simulink model "double_3D_pend"  (R2023a)
settings: Solver=VariableStepAuto  StartTime=0.0  StopTime=5  MaxStep=1e-3  RelTol=1e-9  AbsTol=1e-9  EnableMultiTasking=on
InitFcn:
  | addpath quaternion_muscle\
  | data;
values from neighbouring files (symbols this model uses):
  akt = [1,1,1]    [data.m]    (also in odvozeni_svaly.m = sym('akt',[1 6]); optim_control_nlmpc.m = u'; simulation.m = [1,1,1]*0.5)
  c = 0    [data.m]    (also in neco.m = cos(0); optim_control_nlmpc.m = 100; simulation.m = 10)
  force = [1,1,0]*(-30)    [data.m]    (also in odvozeni_svaly.m = (((length / l0m)^3) * exp(8 * length / l0m - 12.9) + (exp(-(; optim_control_nlmpc.m = [1,1,1,1,1,1]*(30); simulation.m = -[1,2,1]*1)
  g = 9.81    [data.m]    (also in optim_control_nlmpc.m; simulation.m)
  IL = [8.1667, 8.1667, 1.66667,0,0,0]    [data.m]    (also in fo_python_to_matlab.m = [ILxx ILyy ILzz ILxy ILyz ILzx]; mm_python_to_matlab.m = [ILxx ILyy ILzz ILxy ILyz ILzx]; optim_control_nlmpc.m; simulation.m = [84.1667, 84.1667, 1.66667])
  initialConditions = [1,0,0,0,0,0,zeros(1,6)]*2    [data.m]    (also in simulation.m = [1,1,1,1,1,1,0,0,0,0,0,0]*0)
  IU = [8.1667, 8.1667, 1.66667,0,0,0]    [data.m]    (also in fo_python_to_matlab.m = [IUxx IUyy IUzz IUxy IUyz IUzx]; mm_python_to_matlab.m = [IUxx IUyy IUzz IUxy IUyz IUzx]; optim_control_nlmpc.m; simulation.m = [84.1667, 84.1667, 1.66667]*1e-2)
  k = 100    [data.m]    (also in neco.m = elips_pars.k; optim_control_nlmpc.m = 0; simulation.m = 1)
  l0m = [12,25,15]    [data.m]    (also in odvozeni_svaly.m = sym('l0m', [1 6]); optim_control_nlmpc.m = [30,30,30,30,30,30]; simulation.m = [10,20,10])
  m = rand(1,2)*10    [data.m]    (also in fo_python_to_matlab.m = [m1,m2]; mm_python_to_matlab.m = [m1,m2]; neco.m = elips_pars.m; optim_control_nlmpc.m = [5,10])
  rigid1C = [0,0,5]    [data.m]    (also in fo_python_to_matlab.m = [rigid1Cx, rigid1Cy, rigid1Cz]; mm_python_to_matlab.m = [rigid1Cx, rigid1Cy, rigid1Cz]; optim_control_nlmpc.m)
  rigid1P = [0,0,-5]    [data.m]    (also in fo_python_to_matlab.m = [rigid1Px, rigid1Py, rigid1Pz]; mm_python_to_matlab.m = [rigid1Px, rigid1Py, rigid1Pz]; optim_control_nlmpc.m)
  rigid2C = [0,0,5]    [data.m]    (also in fo_python_to_matlab.m = [rigid2Cx, rigid2Cy, rigid2Cz]; mm_python_to_matlab.m = [rigid2Cx, rigid2Cy, rigid2Cz]; optim_control_nlmpc.m)
  s = sin(0)    [neco.m]
undefined symbols (not defined in the file or in its folder): Ixx, Iyy, Izz, l, q1init, q2init, X, Y, Z
libraries: sm_lib x104, nesl_utility x52
(part 4 of 5)

== system double_3D_pend/Subsystem5 ==
  PS-Simulink Converter : nesl_utility/PS-Simulink Converter  PhysicalDomain=network_engine_domain  SubClassName=ps_output  LeftPortType=input  RightPortType=output  PseudoPeriodic=off  Frequencies=[]  VectorFormat=inherit  Unit=inherit  AffineConversion=off
  Spherical Joint1 : sm_lib/Joints/Spherical Joint  JointMode=Normal  SenseConstraintForce=off  SenseConstraintForceX=off  SenseConstraintForceY=off  SenseConstraintForceZ=off  SenseConstraintTorque=off  SenseConstraintTorqueX=off  SenseConstraintTorqueY=off  SenseConstraintTorqueZ=off  SenseTotalForce=off  SenseTotalForceX=off  SenseTotalForceY=off  SenseTotalForceZ=off  SenseTotalTorque=off  SenseTotalTorqueX=off  SenseTotalTorqueY=off  SenseTotalTorqueZ=off  CompositeWrenchDir=FollowerOnBase  CompositeWrenchFrame=BaseFrame  EqPosRotationMethod=None  EqPosRotationAngleUnits=deg  EqPosRotationStandardAxis=+Z  EqPosRotationAngle=0.0  EqPosRotationArbitraryAxis=[0 0 1]  EqPosFollAlignAxisA=+X  EqPosBaseAlignAxisA=+Y  EqPosFollAlignAxisB=+Y  EqPosBaseAlignAxisB=+Z  EqPosRotationSequenceAxes=FollowerAxes  EqPosRotationSequence=XYX  EqPosRotationSequenceAngles=[0 0 0]  EqPosRotationSequenceAnglesUnits=deg  EqPosRotationMatrix=[1 0 0; 0 1 0; 0 0 1]  EqPosQuaternion=[1 0 0 0]  SpringStiffness=0  SpringStiffnessUnits=N*m/deg  DampingCoefficient=c  DampingCoefficientUnits=N*m/(rad/s)  ActuateTorqueX=off  ActuateTorqueY=off  ActuateTorqueZ=off  ActuateTorque=off  TorqueActuationMode=InputTorque  MotionActuationMode=ComputedMotion  ActuationFrame=FollowerFrame  SensePosition=on  SenseVelocityX=off  SenseVelocityY=off  SenseVelocityZ=off  SenseVelocity=off  SenseAccelerationX=off  SenseAccelerationY=off  SenseAccelerationZ=off  SenseAcceleration=off  SenseTorqueX=off  SenseTorqueY=off  SenseTorqueZ=off  SenseTorqueForce=off  SenseLowerLimitTorqueMag=off  SenseUpperLimitTorqueMag=off  SensingFrame=BaseFrame  LowerLimitSpecify=off  LowerLimitBound=15  LowerLimitBoundUnits=deg  LowerLimitStiffness=1e4  LowerLimitStiffnessUnits=N*m/deg  LowerLimitDamping=10  LowerLimitDampingUnits=N*m/(deg/s)  LowerLimitTransitionRegionWidth=0.1  LowerLimitTransitionRegionWidthUnits=deg  UpperLimitSpecify=off  UpperLimitBound=45  UpperLimitBoundUnits=deg  UpperLimitStiffness=1e4  UpperLimitStiffnessUnits=N*m/deg  UpperLimitDamping=10  UpperLimitDampingUnits=N*m/(deg/s)  UpperLimitTransitionRegionWidth=0.1  UpperLimitTransitionRegionWidthUnits=deg  PositionTargetRotationMethod=Quaternion  PositionTargetRotationAngleUnits=deg  PositionTargetRotationStandardAxis=+Z  PositionTargetRotationAngle=0.0  PositionTargetRotationArbitraryAxis=[0 0 1]  PositionTargetFollAlignAxisA=+X  PositionTargetBaseAlignAxisA=+Y  PositionTargetFollAlignAxisB=+Y  PositionTargetBaseAlignAxisB=+Z  PositionTargetRotationSequenceAxes=FollowerAxes  PositionTargetRotationSequence=XYZ  PositionTargetRotationSequenceAngles=initialConditions(4:6)  PositionTargetRotationSequenceAnglesUnits=rad  PositionTargetRotationMatrix=[1 0 0; 0 1 0; 0 0 1]  PositionTargetQuaternion=q2init  PositionTargetSpecify=on  PositionTargetPriority=High  VelocityTargetValue=[0 0 0]  VelocityTargetValueUnits=deg/s  VelocityTargetSpecify=off  VelocityTargetPriority=High  VelocityTargetInFollowerFrame=on
  B : PMIOPort  Side=Left
  F : PMIOPort  Port=2  Side=Right
  Outport : Outport
  wires:
  PS-Simulink Converter/1 -> Outport/1
  connections:
  Spherical Joint1/RConn2 -- PS-Simulink Converter/LConn1
  Spherical Joint1/RConn1 -- F/RConn1
  B/RConn1 -- Spherical Joint1/LConn1

== matlab function double_3D_pend/Transform matrix ==
  data: u input; R output
function R = fcn(u)

R = zeros(3,3);

rot = xyzSeq(u(1),u(2),u(3))*xyzSeq(u(4),u(5),u(6));
R = rot(1:3,1:3);

function xyz = xyzSeq(x,y,z)
    xyz = R_x(x)*R_y(y)*R_z(z);
end
    
function rot_phix = R_x(phix)
    rot_phix = [1,0        , 0        ,0;
                0,cos(phix),-sin(phix),0;
                0,sin(phix), cos(phix),0;
                0,0        , 0        ,1];
end

function rot_phiy = R_y(phiy)
    rot_phiy = [cos(phiy),0,sin(phiy),0;
                0        ,1,0        ,0;
               -sin(phiy),0,cos(phiy),0;
                0        ,0,0        ,1];
end

function rot_phiz = R_z(phiz)
    rot_phiz = [cos(phiz),-sin(phiz),0,0;
                sin(phiz), cos(phiz),0,0;
                0           ,0      ,1,0;
                0           ,0      ,0,1];
end

end

== matlab function double_3D_pend/DELT13/Active_factor_norm ==
  data: Fa_norm output; lm input; l0 input; a input
function Fa_norm = fcn(lm,l0,a)
f_gauss = 0.25;
Fa_norm = (exp(-(lm/l0-1)^2/f_gauss))*a;

== matlab function double_3D_pend/DELT4/Active_factor_norm ==
  data: Fa_norm output; lm input; l0 input; a input
function Fa_norm = fcn(lm,l0,a)
f_gauss = 0.25;
Fa_norm = (exp(-(lm/l0-1)^2/f_gauss))*a;

== matlab function double_3D_pend/DELT4/Passive_force_norm ==
  data: lm input; Fp_norm output; l0 input
function Fp_norm = fcn(lm,l0)
Fp_norm = ((lm/l0)^3)*exp(8*lm/l0-12.9);

== matlab function double_3D_pend/DELT5/Active_factor_norm ==
  data: Fa_norm output; lm input; l0 input; a input
function Fa_norm = fcn(lm,l0,a)
f_gauss = 0.25;
Fa_norm = (exp(-(lm/l0-1)^2/f_gauss))*a;

== matlab function double_3D_pend/DELT5/Passive_force_norm ==
  data: lm input; Fp_norm output; l0 input
function Fp_norm = fcn(lm,l0)
Fp_norm = ((lm/l0)^3)*exp(8*lm/l0-12.9);

== matlab function double_3D_pend/DELT6/Active_factor_norm ==
  data: Fa_norm output; lm input; l0 input; a input
function Fa_norm = fcn(lm,l0,a)
f_gauss = 0.25;
Fa_norm = (exp(-(lm/l0-1)^2/f_gauss))*a;

== matlab function double_3D_pend/DELT6/Passive_force_norm ==
  data: lm input; Fp_norm output; l0 input
function Fp_norm = fcn(lm,l0)
Fp_norm = ((lm/l0)^3)*exp(8*lm/l0-12.9);

== matlab function double_3D_pend/MATLAB Function1 ==
  data: u input; y output
function y = fcn(u)
y = XYZ_angles(u);

== matlab function double_3D_pend/DELT10/Active_factor_norm ==
  data: Fa_norm output; lm input; l0 input; a input
function Fa_norm = fcn(lm,l0,a)
f_gauss = 0.25;
Fa_norm = (exp(-(lm/l0-1)^2/f_gauss))*a;

== matlab function double_3D_pend/DELT10/Passive_force_norm ==
  data: lm input; Fp_norm output; l0 input
function Fp_norm = fcn(lm,l0)
Fp_norm = ((lm/l0)^3)*exp(8*lm/l0-12.9);

== matlab function double_3D_pend/DELT11/Active_factor_norm ==
  data: Fa_norm output; lm input; l0 input; a input
function Fa_norm = fcn(lm,l0,a)
f_gauss = 0.25;
Fa_norm = (exp(-(lm/l0-1)^2/f_gauss))*a;

== matlab function double_3D_pend/DELT11/Passive_force_norm ==
  data: lm input; Fp_norm output; l0 input
function Fp_norm = fcn(lm,l0)
Fp_norm = ((lm/l0)^3)*exp(8*lm/l0-12.9);

== matlab function double_3D_pend/DELT12/Active_factor_norm ==
  data: Fa_norm output; lm input; l0 input; a input
function Fa_norm = fcn(lm,l0,a)
f_gauss = 0.25;
Fa_norm = (exp(-(lm/l0-1)^2/f_gauss))*a;

== matlab function double_3D_pend/DELT12/Passive_force_norm ==
  data: lm input; Fp_norm output; l0 input
function Fp_norm = fcn(lm,l0)
Fp_norm = ((lm/l0)^3)*exp(8*lm/l0-12.9);

== matlab function double_3D_pend/DELT7/Active_factor_norm ==
  data: Fa_norm output; lm input; l0 input; a input
function Fa_norm = fcn(lm,l0,a)
f_gauss = 0.25;
Fa_norm = (exp(-(lm/l0-1)^2/f_gauss))*a;

== matlab function double_3D_pend/DELT7/Passive_force_norm ==
  data: lm input; Fp_norm output; l0 input
function Fp_norm = fcn(lm,l0)
Fp_norm = ((lm/l0)^3)*exp(8*lm/l0-12.9);

== matlab function double_3D_pend/DELT8/Active_factor_norm ==
  data: Fa_norm output; lm input; l0 input; a input
function Fa_norm = fcn(lm,l0,a)
f_gauss = 0.25;
Fa_norm = (exp(-(lm/l0-1)^2/f_gauss))*a;

== matlab function double_3D_pend/DELT8/Passive_force_norm ==
  data: lm input; Fp_norm output; l0 input
function Fp_norm = fcn(lm,l0)
Fp_norm = ((lm/l0)^3)*exp(8*lm/l0-12.9);

== matlab function double_3D_pend/DELT9/Active_factor_norm ==
  data: Fa_norm output; lm input; l0 input; a input
function Fa_norm = fcn(lm,l0,a)
f_gauss = 0.25;
Fa_norm = (exp(-(lm/l0-1)^2/f_gauss))*a;

== matlab function double_3D_pend/DELT9/Passive_force_norm ==
  data: lm input; Fp_norm output; l0 input
function Fp_norm = fcn(lm,l0)
Fp_norm = ((lm/l0)^3)*exp(8*lm/l0-12.9);

== matlab function double_3D_pend/DELT13/Passive_force_norm ==
  data: lm input; Fp_norm output; l0 input
function Fp_norm = fcn(lm,l0)
Fp_norm = ((lm/l0)^3)*exp(8*lm/l0-12.9);

== matlab function double_3D_pend/DELT14/Active_factor_norm ==
  data: Fa_norm output; lm input; l0 input; a input
function Fa_norm = fcn(lm,l0,a)
f_gauss = 0.25;
Fa_norm = (exp(-(lm/l0-1)^2/f_gauss))*a;

== matlab function double_3D_pend/MATLAB Function5 ==
  data: u input; Izz parameter; Iyy parameter; Ixx parameter; g parameter; l parameter; m parameter; y output; q1new output; q2new output; akt input; l0m parameter; force parameter
function [y,q1new,q2new]  = fcn(u,Izz, Iyy, Ixx, g, l, m,akt, l0m, force)
t = 0;
y = zeros(14,1);
q1 = u(1:4);
q2 = u(5:8);

q1m = u(1:4);
q2m = u(5:8);

if q1(1) < 0
    q1m = q1*-1;
end
%
if q2(1) < 0
    q2m = q2*-1;
end

q1newm = q1m/norm(q1m);
q2newm = q2m/norm(q2m);
q1new = q1/norm(q1);
q2new = q2/norm(q2);
u1 = u(9:11);
u2 = u(12:end);
FM = FE_Q_stack(0,[q1newm;q2newm]',force,l0m,akt');
MM = mm_moje(t,[q1new;q2new]',[u1;u2]',Ixx,Iyy,Izz,l,m, g);
FE = fe_moje(t,[q1new;q2new]',[u1;u2]',Ixx,Iyy,Izz,l,m, g);
y = MM\(FE+[zeros(8,1);FM]);

function res = G(Q)
Q0 = Q(1);
Q1 = Q(2);
Q2 = Q(3);
Q3 = Q(4);
res = [-Q1, Q0, Q3, -Q2;
        -Q2,-Q3, Q0, Q1;
        -Q3, Q2, -Q1, Q0];
end
end

== matlab function double_3D_pend/DELT1/Active_factor_norm ==
  data: Fa_norm output; lm input; l0 input; a input
function Fa_norm = fcn(lm,l0,a)
f_gauss = 0.25;
Fa_norm = (exp(-(lm/l0-1)^2/f_gauss))*a;

== matlab function double_3D_pend/DELT14/Passive_force_norm ==
  data: lm input; Fp_norm output; l0 input
function Fp_norm = fcn(lm,l0)
Fp_norm = ((lm/l0)^3)*exp(8*lm/l0-12.9);

== matlab function double_3D_pend/DELT15/Active_factor_norm ==
  data: Fa_norm output; lm input; l0 input; a input
function Fa_norm = fcn(lm,l0,a)
f_gauss = 0.25;
Fa_norm = (exp(-(lm/l0-1)^2/f_gauss))*a;

== matlab function double_3D_pend/DELT15/Passive_force_norm ==
  data: lm input; Fp_norm output; l0 input
function Fp_norm = fcn(lm,l0)
Fp_norm = ((lm/l0)^3)*exp(8*lm/l0-12.9);

== matlab function double_3D_pend/DELT16/Active_factor_norm ==
  data: Fa_norm output; lm input; l0 input; a input
function Fa_norm = fcn(lm,l0,a)
f_gauss = 0.25;
Fa_norm = (exp(-(lm/l0-1)^2/f_gauss))*a;

== matlab function double_3D_pend/DELT16/Passive_force_norm ==
  data: lm input; Fp_norm output; l0 input
function Fp_norm = fcn(lm,l0)
Fp_norm = ((lm/l0)^3)*exp(8*lm/l0-12.9);

== matlab function double_3D_pend/DELT17/Active_factor_norm ==
  data: Fa_norm output; lm input; l0 input; a input
function Fa_norm = fcn(lm,l0,a)
f_gauss = 0.25;
Fa_norm = (exp(-(lm/l0-1)^2/f_gauss))*a;

== matlab function double_3D_pend/DELT17/Passive_force_norm ==
  data: lm input; Fp_norm output; l0 input
function Fp_norm = fcn(lm,l0)
Fp_norm = ((lm/l0)^3)*exp(8*lm/l0-12.9);

== matlab function double_3D_pend/DELT18/Active_factor_norm ==
  data: Fa_norm output; lm input; l0 input; a input
function Fa_norm = fcn(lm,l0,a)
f_gauss = 0.25;
Fa_norm = (exp(-(lm/l0-1)^2/f_gauss))*a;

== matlab function double_3D_pend/DELT18/Passive_force_norm ==
  data: lm input; Fp_norm output; l0 input
function Fp_norm = fcn(lm,l0)
Fp_norm = ((lm/l0)^3)*exp(8*lm/l0-12.9);
